simulink model "Pacemaker_v3"  (R2025a)
settings: Solver=FixedStepAuto  StartTime=0.0  StopTime=10.0  FixedStep=1e-3  RelTol=1e-3  EnableMultiTasking=on
undefined symbols (not defined in the file or in its folder): D0, D1, D10, D11, D12, D13, D2, D3, D4, D5, D6, D7, D8, D9, PTA0, PTA1, PTA2, PTB23, PTB9, PTC16, PTC17, PTC2, PTC3, PTC4, PTD0, PTD1, PTD2, PTD3
libraries: frdmk64flib x17, dspstat3 x3
settings Model: ExtModeTrigDuration=5  Creator=tphil  LastModifiedBy=tphil
settings OptimizationCC: DefaultParameterBehavior=Inlined  EnhancedBackFolding=on  PassReuseOutputArgsAs=Individual arguments  ZeroExternalMemoryAtStartup=off  ZeroInternalMemoryAtStartup=off  MaxStackSize=64  OptimizeBlockOrder=speed  DifferentSizesBufferReuse=on  OptimizationCustomize=off  EfficientTunableParamExpr=on
settings DebuggingCC: ParameterTunabilityLossMsg=error
settings HardwareCC: ProdBitPerPointer=32.0  ProdBitPerSizeT=32.0  ProdBitPerPtrDiffT=32.0  ProdLargestAtomicInteger=Long  ProdLargestAtomicFloat=Double  ProdWordSize=32.0  ProdHWDeviceType=ARM Compatible->ARM Cortex
settings SFSimCC: MATLABDynamicMemAlloc=off
settings RTWCC: SystemTargetFile=ert.tlc  HardwareBoard=NXP FRDM-K64F  TLCOptions="-aInlineSetEventsForThisBaseRateFcn=TLC_FALSE -aSuppressMultiTaskScheduler=TLC_FALSE  -aRateBasedStepFcn=0"  TemplateMakefile=ert_default_tmf  Toolchain=GNU Tools for ARM Embedded Processors  Description=Embedded Coder
settings CodeAppCC: ForceParamTrailComments=on  IgnoreCustomStorageClasses=off  OperatorAnnotations=on  SimulinkDataObjDesc=on  SFDataObjDesc=on  InsertBlockDesc=on
settings ERTTargetCC: ExtModeTransport=4.0  ExtModeStaticAlloc=off  ExtModeMexFile=sendToCommService  ExtModeIntrfLevel=Level1

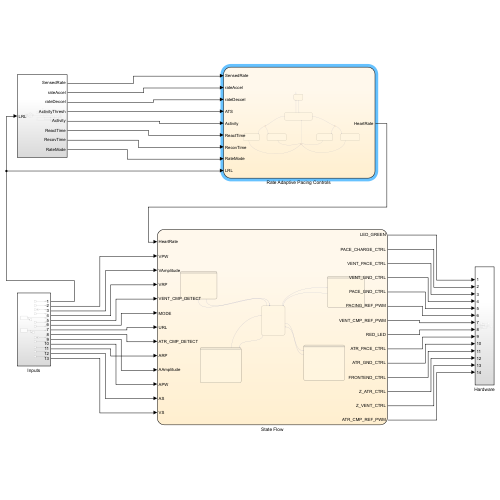
[thumbnail: Simulink's stored preview of the top-level diagram]
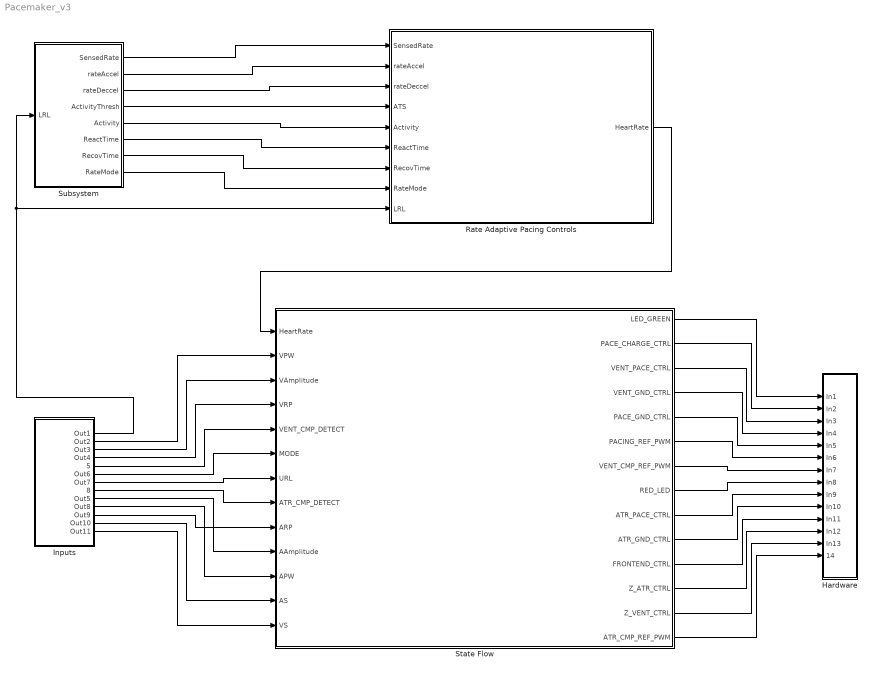
== system Pacemaker_v3 ==
  Hardware : Subsystem
  Inputs : Subsystem
  "Rate Adaptive Pacing Controls " : Stateflow chart  TreatAsAtomicUnit=on
      settings: PortSchema="{\"entries\":[{\"content\":{\"sides\":[{\"content\":{\"connectorIds\":[\"In3\",\"In6\",\"In7\",\"In1\",\"In2\",\"In4\",\"In5\",\"In8\",\"In9\"]},\"type\":\"ConnectorPlacement.EquallySpacedRectSide\",\"uuid\":\"92e350aa-6038-4048-bc49-c80e731bd779\"},{\"content\":{\"connectorIds\":[\"Out1\"],\"side\":\"RIGHT\"},\"type\":\"ConnectorPlacement.EquallySpacedRectSide\",\"uuid\":\"2a0ca1c9-35cf-4a86-8d79-80e737327d0d\"},{\"content\":{\"side\":\"TOP\"},\"type\":\"ConnectorPlacement.EquallySpacedRectSide\",\"uuid\":\"f2a4ce7a-d634-4d9b-abba-ed4089c9553b\"}]},\"type\":\"ConnectorPlacement.EquallySpacedConnector\",\"uuid\":\"812c6488-3371-40ad-aebd-b48230bf77dd\"}],\"packageUris\":[\"http://schema.mathworks.com/mf0/Connector/R2020b\"],\"version\":\"1.0\"}"
  State Flow : Stateflow chart  TreatAsAtomicUnit=on
      settings: PortSchema="{\"entries\":[{\"content\":{\"sides\":[{\"content\":{\"connectorIds\":[\"In13\",\"In1\",\"In2\",\"In3\",\"In4\",\"In5\",\"In6\",\"In7\",\"In8\",\"In9\",\"In10\",\"In11\",\"In12\"]},\"type\":\"ConnectorPlacement.EquallySpacedRectSide\",\"uuid\":\"0070f273-f005-4a83-ad64-757e00c05062\"},{\"content\":{\"connectorIds\":[\"Out1\",\"Out2\",\"Out3\",\"Out4\",\"Out5\",\"Out6\",\"Out7\",\"Out8\",\"Out9\",\"Out10\",\"Out11\",\"Out12\",\"Out13\",\"Out14\"],\"side\":\"RIGHT\"},\"type\":\"ConnectorPlacement.EquallySpacedRectSide\",\"uuid\":\"fe6ab62e-75c4-40d8-bb52-560020ab8d95\"},{\"content\":{\"side\":\"TOP\"},\"type\":\"ConnectorPlacement.EquallySpacedRectSide\",\"uuid\":\"a4f7c297-a2d8-4cb4-bc6f-229f00f06c68\"}]},\"type\":\"ConnectorPlacement.EquallySpacedConnector\",\"uuid\":\"ce088916-88df-45d3-a679-886f8bf7c207\"}],\"packageUris\":[\"http://schema.mathworks.com/mf0/Connector/R2020b\"],\"version\":\"1.0\"}"
  Subsystem : Subsystem
  wires:
  State Flow/13(Z_VENT_CTRL) -> Hardware/13(In13)
  State Flow/2(PACE_CHARGE_CTRL) -> Hardware/2(In2)
  Inputs/3(Out3) -> State Flow/2(VAmplitude)
  State Flow/1(LED_GREEN) -> Hardware/1(In1)
  State Flow/7(VENT_CMP_REF_PWM) -> Hardware/7(In7)
  State Flow/8(RED_LED) -> Hardware/8(In8)
  State Flow/10(ATR_GND_CTRL) -> Hardware/10(In10)
  State Flow/4(VENT_GND_CTRL) -> Hardware/4(In4)
  State Flow/9(ATR_PACE_CTRL) -> Hardware/9(In9)
  Inputs/4(Out4) -> State Flow/3(VRP)
  Inputs/8(8) -> State Flow/7(ATR_CMP_DETECT)
  State Flow/12(Z_ATR_CTRL) -> Hardware/12(In12)
  Inputs/10(Out8) -> State Flow/10(APW)
  Inputs/2(Out2) -> State Flow/1(VPW)
  State Flow/3(VENT_PACE_CTRL) -> Hardware/3(In3)
  State Flow/14(ATR_CMP_REF_PWM) -> Hardware/14(14)
  State Flow/6(PACING_REF_PWM) -> Hardware/6(In6)
  Inputs/13(Out11) -> State Flow/12(VS)
  Inputs/12(Out10) -> State Flow/11(AS)
  Inputs/11(Out9) -> State Flow/8(ARP)
  Inputs/9(Out5) -> State Flow/9(AAmplitude)
  Inputs/7(Out7) -> State Flow/6(URL)
  State Flow/11(FRONTEND_CTRL) -> Hardware/11(In11)
  Inputs/5(5) -> State Flow/4(VENT_CMP_DETECT)
  State Flow/5(PACE_GND_CTRL) -> Hardware/5(In5)
  Inputs/6(Out6) -> State Flow/5(MODE)
  Inputs/1(Out1) -> Subsystem/1(LRL), "Rate Adaptive Pacing Controls "/9(LRL)
  Subsystem/1(SensedRate) -> "Rate Adaptive Pacing Controls "/3(SensedRate)
  Subsystem/2(rateAccel) -> "Rate Adaptive Pacing Controls "/6(rateAccel)
  Subsystem/3(rateDeccel) -> "Rate Adaptive Pacing Controls "/7(rateDeccel)
  Subsystem/4(ActivityThresh) -> "Rate Adaptive Pacing Controls "/1(ATS)
  Subsystem/5(Activity) -> "Rate Adaptive Pacing Controls "/2(Activity)
  Subsystem/6(ReactTime) -> "Rate Adaptive Pacing Controls "/4(ReactTime)
  Subsystem/7(RecovTime) -> "Rate Adaptive Pacing Controls "/5(RecovTime)
  "Rate Adaptive Pacing Controls "/1(HeartRate) -> State Flow/13(HeartRate)
  Subsystem/8(RateMode) -> "Rate Adaptive Pacing Controls "/8(RateMode)

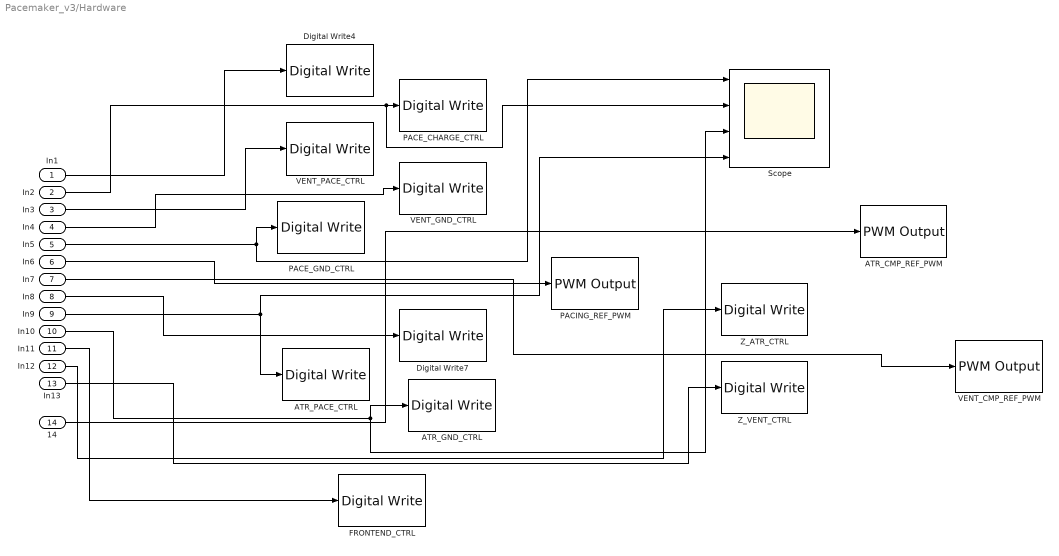
== system Pacemaker_v3/Hardware ==
  In1 : Inport
  In2 : Inport  Port=2
  In3 : Inport  Port=3
  In4 : Inport  Port=4
  In5 : Inport  Port=5
  In6 : Inport  Port=6
  In7 : Inport  Port=7
  In8 : Inport  Port=8
  In9 : Inport  Port=9
  In10 : Inport  Port=10
  In11 : Inport  Port=11
  In12 : Inport  Port=12
  In13 : Inport  Port=13
  14 : Inport  Port=14
  ATR_CMP_REF_PWM : frdmk64flib/PWM Output  Whichpin=PTC2 (D6)  InitialFrequency=2000  InitialDutyCycle=0
  ATR_GND_CTRL : frdmk64flib/Digital Write  Whichpin=PTD2 (D11)
  ATR_PACE_CTRL : frdmk64flib/Digital Write  Whichpin=PTA0 (D8)
  Digital Write4 : frdmk64flib/Digital Write  Whichpin=GREEN_LED
  Digital Write7 : frdmk64flib/Digital Write  Whichpin=RED_LED
  FRONTEND_CTRL : frdmk64flib/Digital Write  Whichpin=PTD1 (D13)
  PACE_CHARGE_CTRL : frdmk64flib/Digital Write  Whichpin=PTB9 (D2)
  PACE_GND_CTRL : frdmk64flib/Digital Write  Whichpin=PTD0 (D10)
  PACING_REF_PWM : frdmk64flib/PWM Output  Whichpin=PTA2 (D5)  InitialFrequency=2000  InitialDutyCycle=30
  Scope : Scope  NumInputPorts=4
      settings: DataLoggingVariableName=ScopeData2
  VENT_CMP_REF_PWM : frdmk64flib/PWM Output  Whichpin=PTA1 (D3)  InitialFrequency=2000  InitialDutyCycle=0
  VENT_GND_CTRL : frdmk64flib/Digital Write  Whichpin=PTD3 (D12)
  VENT_PACE_CTRL : frdmk64flib/Digital Write  Whichpin=PTC4 (D9)
  Z_ATR_CTRL : frdmk64flib/Digital Write  Whichpin=PTB23 (D4)
  Z_VENT_CTRL : frdmk64flib/Digital Write  Whichpin=PTC3 (D7)
  wires:
  In10/1 -> Scope/3, ATR_GND_CTRL/1
  In2/1 -> Scope/2, PACE_CHARGE_CTRL/1
  In6/1 -> PACING_REF_PWM/1
  In4/1 -> VENT_GND_CTRL/1
  In13/1 -> Z_VENT_CTRL/1
  In1/1 -> Digital Write4/1
  In5/1 -> PACE_GND_CTRL/1, Scope/1
  In3/1 -> VENT_PACE_CTRL/1
  In9/1 -> ATR_PACE_CTRL/1, Scope/4
  In8/1 -> Digital Write7/1
  In12/1 -> Z_ATR_CTRL/1
  In11/1 -> FRONTEND_CTRL/1
  14/1 -> ATR_CMP_REF_PWM/1
  In7/1 -> VENT_CMP_REF_PWM/1

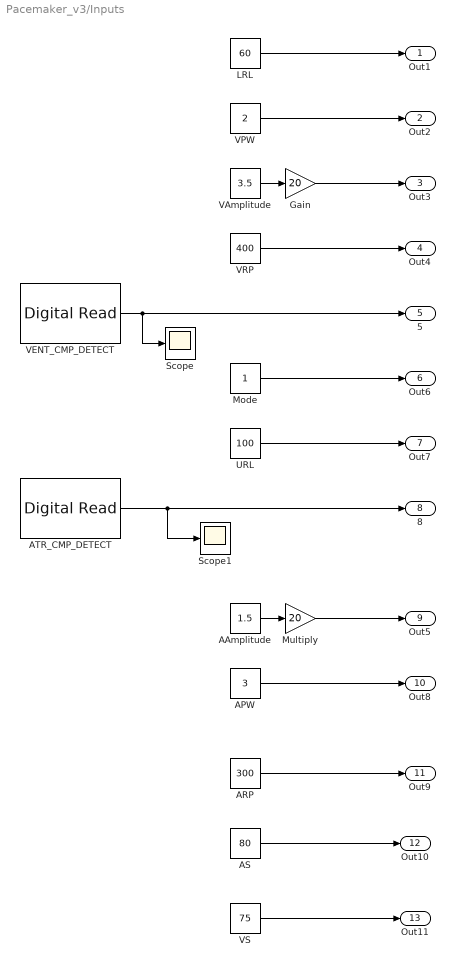
== system Pacemaker_v3/Inputs ==
  AAmplitude : Constant  Value=1.5  OutDataTypeStr=double
  APW : Constant  Value=3  OutDataTypeStr=double
  ARP : Constant  Value=300  OutDataTypeStr=double
  AS : Constant  Value=80  OutDataTypeStr=double
  ATR_CMP_DETECT : frdmk64flib/Digital Read  Whichpin=PTC16 (D0)  SampleTime=-1
  Gain : Gain  Gain=20
  LRL : Constant  Value=60  OutDataTypeStr=double
  Mode : Constant  OutDataTypeStr=int16
  Multiply : Gain  Gain=20
  Scope : Scope
      settings: ActiveDisplayYMinimum=0.9  ActiveDisplayYMaximum=1.1
  Scope1 : Scope
      settings: ActiveDisplayYMinimum=0.9  ActiveDisplayYMaximum=1.1
  URL : Constant  Value=100  OutDataTypeStr=double
  VAmplitude : Constant  Value=3.5  OutDataTypeStr=double
  VENT_CMP_DETECT : frdmk64flib/Digital Read  Whichpin=PTC17 (D1)  SampleTime=inf
  VPW : Constant  Value=2  OutDataTypeStr=double
  VRP : Constant  Value=400  OutDataTypeStr=double
  VS : Constant  Value=75  OutDataTypeStr=double
  Out1 : Outport
  Out2 : Outport  Port=2
  Out3 : Outport  Port=3
  Out4 : Outport  Port=4
  5 : Outport  Port=5
  Out6 : Outport  Port=6
  Out7 : Outport  Port=7
  8 : Outport  Port=8
  Out5 : Outport  Port=9
  Out8 : Outport  Port=10
  Out9 : Outport  Port=11
  Out10 : Outport  Port=12
  Out11 : Outport  Port=13
  wires:
  VPW/1 -> Out2/1
  VAmplitude/1 -> Gain/1
  VENT_CMP_DETECT/1 -> 5/1, Scope/1
  VRP/1 -> Out4/1
  Mode/1 -> Out6/1
  LRL/1 -> Out1/1
  Gain/1 -> Out3/1
  URL/1 -> Out7/1
  ATR_CMP_DETECT/1 -> Scope1/1, 8/1
  AAmplitude/1 -> Multiply/1
  Multiply/1 -> Out5/1
  APW/1 -> Out8/1
  ARP/1 -> Out9/1
  AS/1 -> Out10/1
  VS/1 -> Out11/1

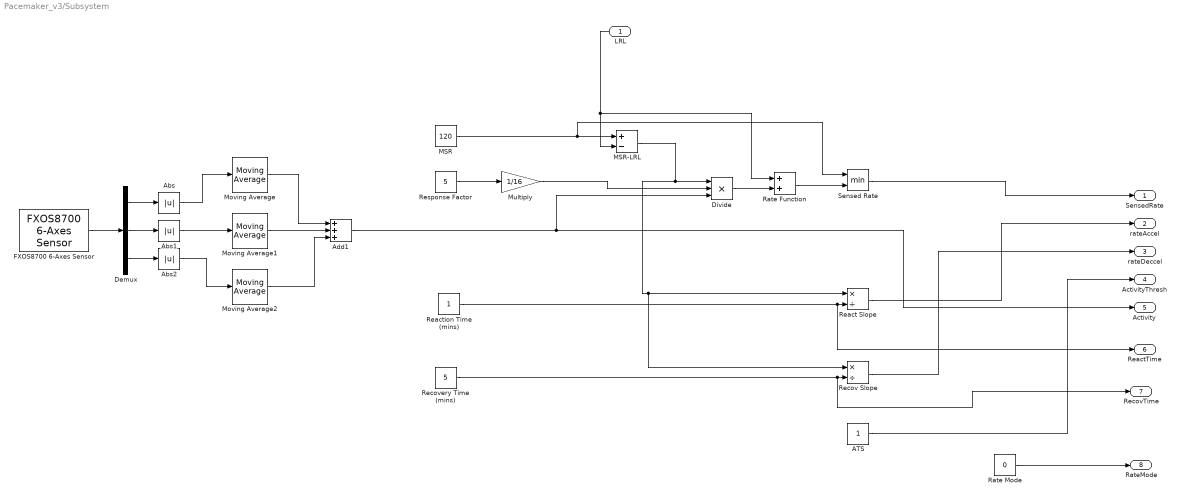
== system Pacemaker_v3/Subsystem ==
  LRL : Inport
  ATS : Constant  OutDataTypeStr=double
  Abs : Abs  SaturateOnIntegerOverflow=off
  Abs1 : Abs  SaturateOnIntegerOverflow=off
  Abs2 : Abs  SaturateOnIntegerOverflow=off
  Add1 : Sum  Inputs=+++
  Demux : Demux  Outputs=3
  Divide : Product  Inputs=***
  FXOS8700 6-Axes Sensor : frdmk64flib/FXOS8700 6-Axes Sensor  Activesensor=Accelerometer only  ODR=800Hz  HybridODR=400Hz  Accelfullrange=-4g to +4g  SampleTime=-1
  MSR : Constant  Value=120  OutDataTypeStr=double
  MSR-LRL : Sum  Inputs=+-
  Moving Average : dspstat3/Moving Average  Method=Sliding window  ForgettingFactorPort=off  SpecifyWindowLength=on  WindowLength=900  OverlapLength=899  AllowArbitraryInputLength=off  ForgettingFactor=0.9  SimulateUsing=Interpreted execution
  Moving Average1 : dspstat3/Moving Average  Method=Sliding window  ForgettingFactorPort=off  SpecifyWindowLength=on  WindowLength=900  OverlapLength=899  AllowArbitraryInputLength=off  ForgettingFactor=0.9  SimulateUsing=Interpreted execution
  Moving Average2 : dspstat3/Moving Average  Method=Sliding window  ForgettingFactorPort=off  SpecifyWindowLength=on  WindowLength=900  OverlapLength=899  AllowArbitraryInputLength=off  ForgettingFactor=0.9  SimulateUsing=Interpreted execution
  Multiply : Gain  Gain=1/16
  Rate Function : Sum
  Rate Mode : Constant  Value=0
  React Slope : Product  Inputs=*/  OutDataTypeStr=double
  "Reaction Time (mins) " : Constant  OutDataTypeStr=double
  Recov Slope : Product  Inputs=*/  OutDataTypeStr=double
  Recovery Time (mins) : Constant  Value=5  OutDataTypeStr=double
  Response Factor : Constant  Value=5  OutDataTypeStr=double
  Sensed Rate : MinMax  Inputs=2
  SensedRate : Outport
  rateAccel : Outport  Port=2
  rateDeccel : Outport  Port=3
  ActivityThresh : Outport  Port=4
  Activity : Outport  Port=5
  ReactTime : Outport  Port=6
  RecovTime : Outport  Port=7
  RateMode : Outport  Port=8
  wires:
  Recovery Time (mins)/1 -> RecovTime/1, Recov Slope/2
  Demux/3 -> Abs2/1
  LRL/1 -> Rate Function/1, MSR-LRL/2
  FXOS8700 6-Axes Sensor/1 -> Demux/1
  Abs2/1 -> Moving Average2/1
  Rate Function/1 -> Sensed Rate/2
  Demux/2 -> Abs1/1
  Demux/1 -> Abs/1
  Moving Average2/1 -> Add1/3
  MSR-LRL/1 -> Recov Slope/1, React Slope/1, Divide/1
  Moving Average1/1 -> Add1/2
  Abs/1 -> Moving Average/1
  Abs1/1 -> Moving Average1/1
  Divide/1 -> Rate Function/2
  "Reaction Time (mins) "/1 -> ReactTime/1, React Slope/2
  Moving Average/1 -> Add1/1
  Response Factor/1 -> Multiply/1
  Multiply/1 -> Divide/2
  MSR/1 -> Sensed Rate/1, MSR-LRL/1
  Sensed Rate/1 -> SensedRate/1
  ATS/1 -> ActivityThresh/1
  React Slope/1 -> rateAccel/1
  Recov Slope/1 -> rateDeccel/1
  Rate Mode/1 -> RateMode/1
  Add1/1 -> Activity/1, Divide/3

== stateflow chart Pacemaker_v3/Rate Adaptive Pacing Controls  ==
  state INIT
    entry:
    HeartRate = LRL;
    noactTime = 0;
    actTime = 0;
  state CheckActivity
    entry:
    actPeriod = 1/(LRL+(SensedRate-LRL)*actTime/ReactTime);
    noactPeriod = 1/(LRL+(SensedRate-LRL)*noactTime/RecovTime);
    actTime = actTime + actPeriod;
    noactTime = noactTime + noactPeriod;
  state AtSensedRate
    entry:
    HeartRate = SensedRate;
    actTime = 0;
  state IncreaseHeartRate
    entry:
    HeartRate = HeartRate + rateAccel*actTime;
  state AtLRL
    entry:
    HeartRate = LRL;
  state DecreaseHeartRate
    entry:
    HeartRate = HeartRate - rateDeccel*noactTime;
    noactTime = 0;
  (default) -> INIT
  CheckActivity -> INIT [order 2] : [RateMode == 0]
  INIT -> CheckActivity : [RateMode == 1]
  CheckActivity -> (junction 24) [order 1] : [Activity>ATS]
  CheckActivity -> (junction 25) [order 3] : [Activity<ATS]
  (junction 38) -> CheckActivity
  (junction 25) -> DecreaseHeartRate [order 2]
  (junction 24) -> AtSensedRate [order 1] : [HeartRate + rateAccel*actTime >= SensedRate]
  (junction 25) -> AtLRL [order 1] : [HeartRate - rateDeccel*noactTime <= LRL]
  (junction 24) -> IncreaseHeartRate [order 2]
  AtSensedRate -> (junction 38)
  IncreaseHeartRate -> (junction 38)
  DecreaseHeartRate -> (junction 38)
  AtLRL -> (junction 38)
  data: ATS input double; Activity input double; SensedRate input double; ReactTime input double; RecovTime input double; rateAccel input double; rateDeccel input double; RateMode input; HeartRate output; LRL input double; noactTime local double; actTime local double; actPeriod local double; noactPeriod local double

== stateflow chart Pacemaker_v3/State Flow ==
  state AOOX
    entry:
    % Initialize PACE_GND_CTRL and set the PWM amplitude to the Atrial Amplitude
    PACE_GND_CTRL = 1;
    PACING_REF_PWM = VAmplitude;
    state TIMING
      entry:
      % upon entry into AOO send no pulse
      % and wait for a period - the APW
      LED_GREEN = 0;
      ATR_PACE_CTRL = 0;
      PACE_CHARGE_CTRL =1;
      ATR_GND_CTRL = 1;
    state PULSE
      entry:
      % after set duration has passed, send
      % a pulse for the APW duration
      LED_GREEN = 1;
      PACE_CHARGE_CTRL =0;
      ATR_GND_CTRL = 0;
      ATR_PACE_CTRL = 1;
    (default) -> AOOX.TIMING
    AOOX.TIMING -> AOOX.PULSE : after(60000/HeartRate -APW, msec)
    AOOX.PULSE -> AOOX.TIMING : after(APW, msec)
  state VOOX
    entry:
    % Initialize PACE_GND_CTRL and set the PWM amplitude to the Ventricular Amplitude
    PACE_GND_CTRL = 1;
    PACING_REF_PWM = VAmplitude;
    state TIMING
      entry:
      % upon entry into VOO send no pulse
      % and wait for a period - the VPW
      LED_GREEN = 0;
      VENT_PACE_CTRL = 0;
      PACE_CHARGE_CTRL =1;
      VENT_GND_CTRL = 1;
    state PULSE
      entry:
      % upon entry into VOO send no pulse
      % and wait for a period - the VPW
      LED_GREEN = 1;
      PACE_CHARGE_CTRL =0;
      VENT_PACE_CTRL = 1;
      VENT_GND_CTRL = 0;
    (default) -> VOOX.TIMING
    VOOX.PULSE -> VOOX.TIMING : after(VPW, msec)
    VOOX.TIMING -> VOOX.PULSE : after(60000/HeartRate-VPW, msec)
  state INITIALIZE
    entry:
    % Initialize inputs
    PACE_CHARGE_CTRL = 0;
    ATR_PACE_CTRL = 0;
    VENT_PACE_CTRL = 0;
    PACE_GND_CTRL = 1;
    ATR_GND_CTRL = 0;
    VENT_GND_CTRL=0;
    FRONTEND_CTRL=1;
    Z_ATR_CTRL = 0;
    Z_VENT_CTRL=0;
  state VVIX
    entry:
    % set PACE_GND_CTRL to 1 and the PWM amplitude to Ventricular Amplitude
    PACE_GND_CTRL = 1;
    PACING_REF_PWM = VAmplitude;
    % Set the ATR_CMP_REF_PWM to Ventricular sensitivity
    VENT_CMP_REF_PWM=VS;
    state PACE
      entry:
      % if no signal was sensed send pulse
      PACE_CHARGE_CTRL = 0;
      Z_VENT_CTRL=0;
      VENT_PACE_CTRL = 1;
      VENT_GND_CTRL = 0;
      RED_LED = 0;
      LED_GREEN = 1;
    state WAIT
      entry:
      % upon entry wait for signal to be
      % sensed or duration of no pulse
      % to pass
      PACE_CHARGE_CTRL = 1;
      Z_VENT_CTRL=1;
      VENT_PACE_CTRL = 0;
      VENT_GND_CTRL =1;
      RED_LED = 0;
      LED_GREEN = 0;
    state REFRACTORY
      entry:
      % if signal was sensed or VPW duration passed
      % wait for VRP duration and go to WAIT state
      PACE_CHARGE_CTRL = 1;
      Z_VENT_CTRL=1;
      VENT_PACE_CTRL = 0;
      VENT_GND_CTRL = 1;
      RED_LED = 1;
      LED_GREEN = 0;
    (default) -> VVIX.WAIT
    VVIX.WAIT -> VVIX.PACE [order 1] : after(60000/HeartRate -(VPW+VRP), msec)
    VVIX.PACE -> VVIX.REFRACTORY : after(VPW,msec)
    VVIX.WAIT -> VVIX.REFRACTORY [order 2] : [VENT_CMP_DETECT==1]
    VVIX.REFRACTORY -> VVIX.WAIT : after(VRP, msec)
  state AAIX
    entry:
    % set PACE_GND_CTRL to 1 and the PWM amplitude to Atrial Amplitude
    PACE_GND_CTRL = 1;
    PACING_REF_PWM = AAmplitude;
    % Set the ATR_CMP_REF_PWM to Atrial sensitivity
    ATR_CMP_REF_PWM=AS;
    state PACE
      entry:
      % if no signal was sensed send pulse
      PACE_CHARGE_CTRL = 0;
      ATR_PACE_CTRL = 1;
      ATR_GND_CTRL = 0;
      RED_LED = 0;
      LED_GREEN = 1;
    state WAIT
      entry:
      % upon entry wait for signal to be
      % sensed or duration of no pulse
      % to pass
      PACE_CHARGE_CTRL = 1;
      ATR_PACE_CTRL = 0;
      ATR_GND_CTRL =1;
      RED_LED = 0;
      LED_GREEN = 0;
    state REFRACTORY
      entry:
      % if signal was sensed or APW duration passed
      % wait for ARP duration and go to WAIT state
      PACE_CHARGE_CTRL = 1;
      ATR_PACE_CTRL = 0;
      ATR_GND_CTRL = 1;
      RED_LED = 1;
      LED_GREEN = 0;
    (default) -> AAIX.WAIT
    AAIX.WAIT -> AAIX.PACE [order 1] : after(60000/HeartRate -(APW+ARP), msec)
    AAIX.PACE -> AAIX.REFRACTORY : after(APW,msec)
    AAIX.WAIT -> AAIX.REFRACTORY [order 2] : [ATR_CMP_DETECT==1]
    AAIX.REFRACTORY -> AAIX.WAIT : after(ARP, msec)
  INITIALIZE -> VOOX [order 2] : [MODE==2]
  VOOX -> INITIALIZE : [MODE~=2]
  AOOX -> INITIALIZE : [MODE~=1]
  INITIALIZE -> AOOX [order 1] : [MODE==1]
  (default) -> INITIALIZE
  AAIX -> INITIALIZE : [MODE~=4]
  INITIALIZE -> VVIX [order 4] : [MODE==3]
  VVIX -> INITIALIZE : [MODE~=3]
  INITIALIZE -> AAIX [order 3] : [MODE==4]
  data: VPW input double; LED_GREEN output int16; PACE_CHARGE_CTRL output int16; VENT_PACE_CTRL output int16; VENT_GND_CTRL output int16; PACE_GND_CTRL output int16; PACING_REF_PWM output double; VAmplitude input double; VRP input double; VENT_CMP_DETECT input boolean; MODE input int16; VENT_CMP_REF_PWM output; RED_LED output; ATR_PACE_CTRL output; ATR_GND_CTRL output; FRONTEND_CTRL output; Z_ATR_CTRL output; Z_VENT_CTRL output; URL input; ATR_CMP_DETECT input; ATR_CMP_REF_PWM output; ARP input double; AAmplitude input double; APW input double; AS input double; VS input double; HeartRate input
